simulink model "mfbDoubleSoln"  (R2020b)
settings: Solver=VariableStepAuto  StartTime=0.0  StopTime=10.0  RelTol=1e-3
settings Model: Creator=Rocksmithed  LastModifiedBy=Rocksmithed

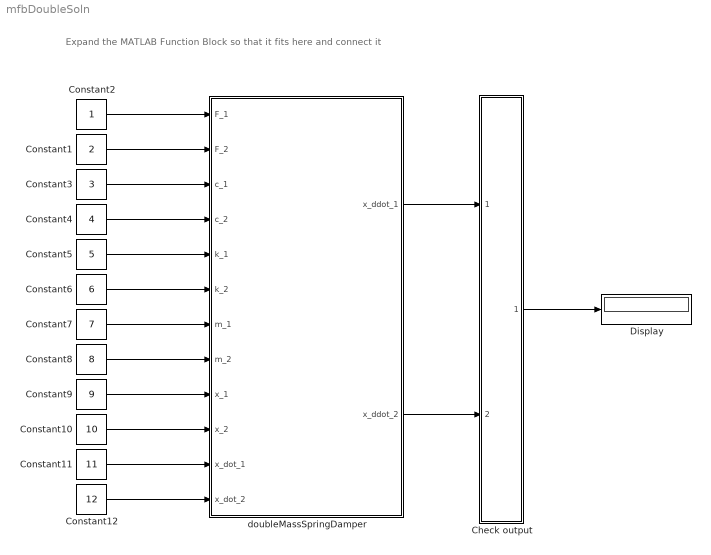
== system mfbDoubleSoln ==
  note: Expand the MATLAB Function Block so that it fits here and connect it
  Check output : Subsystem
  Constant1 : Constant  Value=2
  Constant10 : Constant  Value=10
  Constant11 : Constant  Value=11
  Constant12 : Constant  Value=12
  Constant2 : Constant
  Constant3 : Constant  Value=3
  Constant4 : Constant  Value=4
  Constant5 : Constant  Value=5
  Constant6 : Constant  Value=6
  Constant7 : Constant  Value=7
  Constant8 : Constant  Value=8
  Constant9 : Constant  Value=9
  Display : Display
  doubleMassSpringDamper : MATLAB Function  TreatAsAtomicUnit=on
  wires:
  Constant2/1 -> doubleMassSpringDamper/1(F_1)
  Constant1/1 -> doubleMassSpringDamper/2(F_2)
  Constant3/1 -> doubleMassSpringDamper/3(c_1)
  Constant4/1 -> doubleMassSpringDamper/4(c_2)
  Constant5/1 -> doubleMassSpringDamper/5(k_1)
  Constant6/1 -> doubleMassSpringDamper/6(k_2)
  Constant7/1 -> doubleMassSpringDamper/7(m_1)
  Constant8/1 -> doubleMassSpringDamper/8(m_2)
  Constant9/1 -> doubleMassSpringDamper/9(x_1)
  Constant10/1 -> doubleMassSpringDamper/10(x_2)
  Constant11/1 -> doubleMassSpringDamper/11(x_dot_1)
  Constant12/1 -> doubleMassSpringDamper/12(x_dot_2)
  doubleMassSpringDamper/2(x_ddot_2) -> Check output/2(xddot2)
  Check output/1(Out1) -> Display/1
  doubleMassSpringDamper/1(x_ddot_1) -> Check output/1(xddot1)

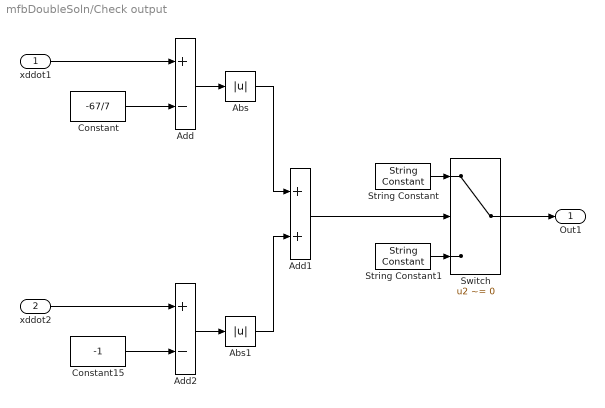
== system mfbDoubleSoln/Check output ==
  xddot1 : Inport
  xddot2 : Inport  Port=2
  Abs : Abs
  Abs1 : Abs
  Add : Sum  Inputs=+-
  Add1 : Sum
  Add2 : Sum  Inputs=+-
  Constant : Constant  Value=-67/7
  Constant15 : Constant  Value=-1
  String Constant : StringConstant  String="\"Incorrect\""
  String Constant1 : StringConstant  String="\"Correct\""
  Switch : Switch  Criteria=u2 ~= 0
  Out1 : Outport
  wires:
  Constant15/1 -> Add2/2
  Constant/1 -> Add/2
  String Constant1/1 -> Switch/3
  Abs/1 -> Add1/1
  Add2/1 -> Abs1/1
  Abs1/1 -> Add1/2
  Add/1 -> Abs/1
  xddot2/1 -> Add2/1
  String Constant/1 -> Switch/1
  xddot1/1 -> Add/1
  Switch/1 -> Out1/1
  Add1/1 -> Switch/2

== matlab function mfbDoubleSoln/doubleMassSpringDamper ==
  data: F_1 input; x_ddot_1 output; F_2 input; c_1 input; c_2 input; k_1 input; k_2 input; m_1 input; m_2 input; x_1 input; x_2 input; x_dot_1 input; x_dot_2 input; x_ddot_2 output
function [x_ddot_1,x_ddot_2] = doubleMassSpringDamper(F_1,F_2,c_1,c_2,k_1,k_2,m_1,m_2,x_1,x_2,x_dot_1,x_dot_2)
%#codegen

%    This function was generated by the Symbolic Math Toolbox version 8.6.
%    19-Nov-2020 15:46:02

x_ddot_1 = -(-F_1+c_1.*x_dot_1+k_1.*x_1+c_2.*(x_dot_1-x_dot_2)+k_2.*(x_1-x_2))./m_1;
if nargout > 1
    x_ddot_2 = (F_2+c_2.*(x_dot_1-x_dot_2)+k_2.*(x_1-x_2))./m_2;
end
